simulink model "practica22022A"  (R2022a)
settings: Solver=FixedStepDiscrete  StartTime=0.0  StopTime=3  FixedStep=0.001  RelTol=1e-3
settings Model: Creator=edgar  LastModifiedBy=Anahi Monserrat
settings ModelReferenceCC: EnableRefExpFcnMdlSchedulingChecks=off
settings RTWCC: Description=Generic Real-Time Target

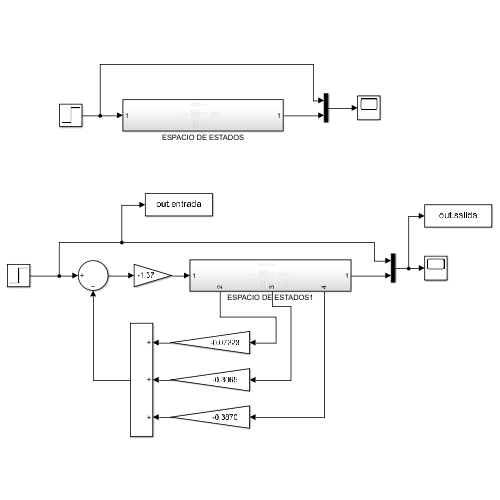
[thumbnail: Simulink's stored preview of the top-level diagram]
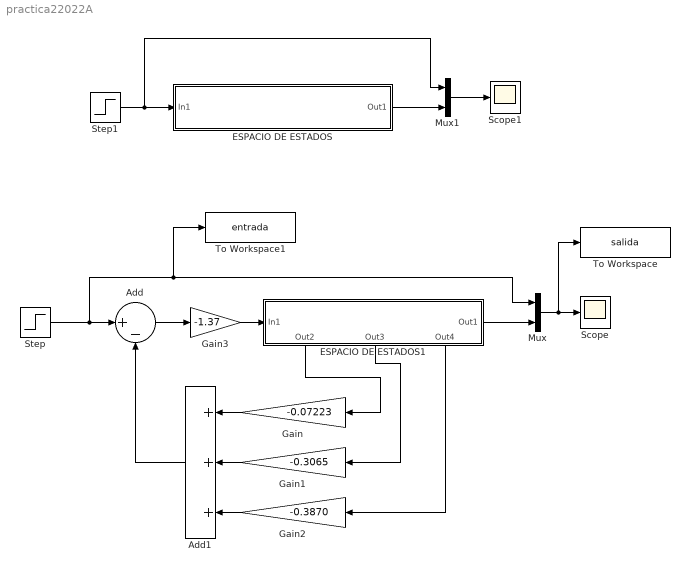
== system practica22022A ==
  Add : Sum  Inputs=|+-
  Add1 : Sum  Inputs=+++
  ESPACIO DE ESTADOS : Subsystem
  ESPACIO DE ESTADOS1 : Subsystem
      settings: PortSchema="{\"entries\":[{\"content\":{\"sides\":[{\"content\":{\"connectorIds\":[\"In1\"]},\"type\":\"ConnectorPlacement.EquallySpacedRectSide\",\"uuid\":\"e4c7e91e-e27a-4516-8912-0ffb8324b1cf\"},{\"content\":{\"connectorIds\":[\"Out1\"],\"side\":\"RIGHT\"},\"type\":\"ConnectorPlacement.EquallySpacedRectSide\",\"uuid\":\"c8b6f25f-762c-42f8-84b8-6d4e17a9e409\"},{\"content\":{\"connectorIds\":[],\"side\":\"TOP\"},\"type\":\"ConnectorPlacement.EquallySpacedRectSide\",\"uuid\":\"20a6fbcd-96ab-4412-bae7-78daeec6f97a\"},{\"content\":{\"connectorIds\":[\"Out2\",\"Out3\",\"Out4\"],\"side\":\"BOTTOM\"},\"type\":\"ConnectorPlacement.EquallySpacedRectSide\",\"uuid\":\"214e34fb-e27d-4adf-9fcb-27d6061738d6\"}]},\"type\":\"ConnectorPlacement.EquallySpacedConnector\",\"uuid\":\"46eb5afa-d204-4a9b-9a44-848bb687e783\"}],\"packageUris\":[\"http://schema.mathworks.com/mf0/Connector/R2020b\"],\"version\":\"1.0\"}"
  Gain : Gain  Gain=-0.07223
  Gain1 : Gain  Gain=-0.3065
  Gain2 : Gain  Gain=-0.3870
  Gain3 : Gain  Gain=-1.37
  Mux : Mux  Inputs=2
  Mux1 : Mux  Inputs=2
  Scope : Scope
  Scope1 : Scope
  Step : Step  SampleTime=0
  Step1 : Step  SampleTime=0
  To Workspace : ToWorkspace  VariableName=salida  SaveFormat=Timeseries  SampleTime=-1
  To Workspace1 : ToWorkspace  VariableName=entrada  SaveFormat=Timeseries  SampleTime=-1
  wires:
  Add/1 -> Gain3/1
  Gain2/1 -> Add1/3
  Gain1/1 -> Add1/2
  Gain/1 -> Add1/1
  Add1/1 -> Add/2
  Mux/1 -> To Workspace/1, Scope/1
  Step/1 -> To Workspace1/1, Mux/1, Add/1
  Gain3/1 -> ESPACIO DE ESTADOS1/1(In1)
  Step1/1 -> Mux1/1, ESPACIO DE ESTADOS/1(In1)
  ESPACIO DE ESTADOS/1(Out1) -> Mux1/2
  Mux1/1 -> Scope1/1
  ESPACIO DE ESTADOS1/2(Out2) -> Gain/1
  ESPACIO DE ESTADOS1/3(Out3) -> Gain1/1
  ESPACIO DE ESTADOS1/4(Out4) -> Gain2/1
  ESPACIO DE ESTADOS1/1(Out1) -> Mux/2

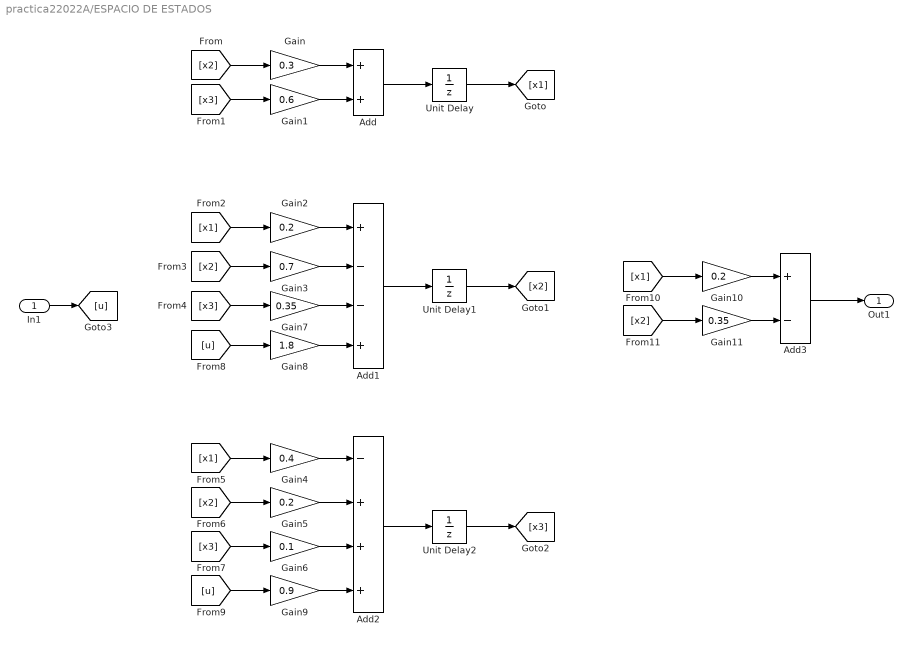
== system practica22022A/ESPACIO DE ESTADOS ==
  In1 : Inport
  Add : Sum
  Add1 : Sum  Inputs=+--+
  Add2 : Sum  Inputs=-+++
  Add3 : Sum  Inputs=+-
  Gain : Gain  Gain=0.3
  Gain1 : Gain  Gain=0.6
  Gain10 : Gain  Gain=0.2
  Gain11 : Gain  Gain=0.35
  Gain2 : Gain  Gain=0.2
  Gain3 : Gain  Gain=0.7
  Gain4 : Gain  Gain=0.4
  Gain5 : Gain  Gain=0.2
  Gain6 : Gain  Gain=0.1
  Gain7 : Gain  Gain=0.35
  Gain8 : Gain  Gain=1.8
  Gain9 : Gain  Gain=0.9
  Unit Delay : UnitDelay  SampleTime=-1  HasFrameUpgradeWarning=on
  Unit Delay1 : UnitDelay  SampleTime=-1  HasFrameUpgradeWarning=on
  Unit Delay2 : UnitDelay  SampleTime=-1  HasFrameUpgradeWarning=on
  Out1 : Outport
  wires:
  Unit Delay/1 -> [x1]
  Unit Delay1/1 -> [x2]
  Unit Delay2/1 -> [x3]
  Add2/1 -> Unit Delay2/1
  Add1/1 -> Unit Delay1/1
  Add/1 -> Unit Delay/1
  Gain/1 -> Add/1
  Gain1/1 -> Add/2
  Gain7/1 -> Add1/3
  Gain3/1 -> Add1/2
  Gain2/1 -> Add1/1
  Gain5/1 -> Add2/2
  Gain4/1 -> Add2/1
  Gain6/1 -> Add2/3
  [x2] -> Gain/1
  [x3] -> Gain1/1
  [x1] -> Gain2/1
  [x2] -> Gain3/1
  [x3] -> Gain7/1
  [x1] -> Gain4/1
  [x2] -> Gain5/1
  [x3] -> Gain6/1
  In1/1 -> [u]
  Gain9/1 -> Add2/4
  [u] -> Gain9/1
  [u] -> Gain8/1
  Gain8/1 -> Add1/4
  Add3/1 -> Out1/1
  [x2] -> Gain11/1
  [x1] -> Gain10/1
  Gain11/1 -> Add3/2
  Gain10/1 -> Add3/1

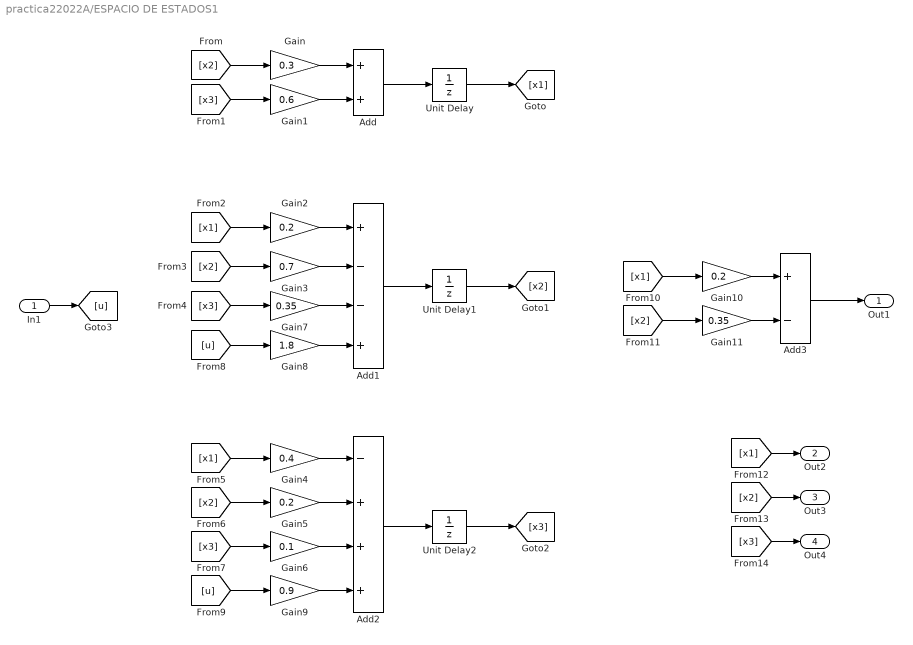
== system practica22022A/ESPACIO DE ESTADOS1 ==
  In1 : Inport
  Add : Sum
  Add1 : Sum  Inputs=+--+
  Add2 : Sum  Inputs=-+++
  Add3 : Sum  Inputs=+-
  Gain : Gain  Gain=0.3
  Gain1 : Gain  Gain=0.6
  Gain10 : Gain  Gain=0.2
  Gain11 : Gain  Gain=0.35
  Gain2 : Gain  Gain=0.2
  Gain3 : Gain  Gain=0.7
  Gain4 : Gain  Gain=0.4
  Gain5 : Gain  Gain=0.2
  Gain6 : Gain  Gain=0.1
  Gain7 : Gain  Gain=0.35
  Gain8 : Gain  Gain=1.8
  Gain9 : Gain  Gain=0.9
  Unit Delay : UnitDelay  SampleTime=-1  HasFrameUpgradeWarning=on
  Unit Delay1 : UnitDelay  SampleTime=-1  HasFrameUpgradeWarning=on
  Unit Delay2 : UnitDelay  SampleTime=-1  HasFrameUpgradeWarning=on
  Out1 : Outport
  Out2 : Outport  Port=2
  Out3 : Outport  Port=3
  Out4 : Outport  Port=4
  wires:
  Gain10/1 -> Add3/1
  Gain11/1 -> Add3/2
  [x1] -> Gain10/1
  [x2] -> Gain11/1
  Add3/1 -> Out1/1
  Gain8/1 -> Add1/4
  [u] -> Gain8/1
  [u] -> Gain9/1
  Gain9/1 -> Add2/4
  In1/1 -> [u]
  [x3] -> Gain6/1
  [x2] -> Gain5/1
  [x1] -> Gain4/1
  [x3] -> Gain7/1
  [x2] -> Gain3/1
  [x1] -> Gain2/1
  [x3] -> Gain1/1
  [x2] -> Gain/1
  Gain6/1 -> Add2/3
  Gain4/1 -> Add2/1
  Gain5/1 -> Add2/2
  Gain2/1 -> Add1/1
  Gain3/1 -> Add1/2
  Gain7/1 -> Add1/3
  Gain1/1 -> Add/2
  Gain/1 -> Add/1
  Add/1 -> Unit Delay/1
  Add1/1 -> Unit Delay1/1
  Add2/1 -> Unit Delay2/1
  Unit Delay2/1 -> [x3]
  Unit Delay1/1 -> [x2]
  Unit Delay/1 -> [x1]
  [x1] -> Out2/1
  [x2] -> Out3/1
  [x3] -> Out4/1
